simulink model "AUAV_V3_TestSensors"  (R2015a)
settings: Solver=FixedStepDiscrete  StartTime=0.0  StopTime=10.0  FixedStep=T  RelTol=1e-3
PreLoadFcn:
  | %T = 0.0025;
  | MavlinkBus;
  | mcuInit;
  | % Baro Altitude Computation
  | % =========================
  | basePressure = 98192.64;
  | baseTemp = 288.215;
  | lapseRate = -0.00198122;
  | baseHeight = 0;
values from neighbouring files (symbols this model uses):
  apSampleTime = 0.01    [mcuInit.m]
  latlong_WP = 1    [mcuInit.m]
  mavlink_attitude_t = Simulink.Bus    [MavlinkBusMarcello.m]
  mavlink_gps_raw_int_t = Simulink.Bus    [MavlinkBus.m]    (also in MavlinkBusMarcello.m)
  mavlink_raw_imu_t = Simulink.Bus    [MavlinkBus.m]    (also in MavlinkBusMarcello.m)
  mavlink_scaled_pressure_t = Simulink.Bus    [MavlinkBus.m]    (also in MavlinkBusMarcello.m)
  mavlink_servo_output_raw_t = Simulink.Bus    [MavlinkBusMarcello.m]
  mavlink_slugs_navigation_t = Simulink.Bus    [MavlinkBusMarcello.m]
  mavlink_sys_status_t = Simulink.Bus    [MavlinkBus.m]    (also in MavlinkBusMarcello.m)
  T = 0.01    [mcuInit.m]
  Xpoints = [0 0]    [mcuInit.m]
  Ypoints = [0 0]    [mcuInit.m]
  Zpoints = [0 0]    [mcuInit.m]
undefined symbols (not defined in the file or in its folder): A0, A14, A15, A2, A3, A4, A5, A6, accBiasRateLimit, B0, bankCommandLimit, barAdjust, baroCutoff, baroCutTemp, cubeAccelGain16405, cubeGyroGain16405, cubeMagGain16405, D0, D11, D7, D8, daLimit, data, daTrimMax, daTrimMin, deLimit, deTrimMax, deTrimMin, drLimit, drTrimMax, drTrimMin, dtLimit, dtTrimMax, dtTrimMin, F2, F3, G0, G13, G15, gaind, GS_location, gyroBiasRateLimit, IC1max, IPStar, ISA_g, Max, maxAcc, MaxDwnPthStar, maxDynPressure, maxEta, mlParamInterface, ms, OC1max, P112, P125, P127, P16, P20, P21, P30 ... (+26)
undefined symbols (not defined in the file): baroOffset, baroScale, barTGain1, barTGain2, barTMean1, barTMean2, bda, bde, bdr, bdt, bICda, bICde, bICdr, bICdt, derivativesConstant, lowRateSensorCutoff, mainSensorCutoff, mda, mde, mdr, mdt, mICda, mICde, mICdr, mICdt, pitotOffset, pitotScale, pitTGain1, pitTGain2, pitTMean1, pitTMean2, powerOffset, powerScale, pressureSensorCutoff, tempOffset, tempScale, vzCutoff, xCutoff, yCutoff
libraries: MCHP_Blockset x158, simulink x84, SLUGS_Library x31, aerolibconvert2 x6, aerolibutil x4, aerolibtransform2 x3, dspmtrx3 x2, aerolibobsolete x2
(part 22 of 24)

== system AUAV_V3_TestSensors/Inner Loop// Navigation/Lateral Channel Encaps [updated 4.28.16]/Lateral Channel/Roll Control [PID]/Trapezoidal Integrator/Protect NaNs  ==
  In1 : Inport
  Integer Delay3 : Delay  DelayLength=1  InputProcessing=Inherited  SampleTime=T
  Relational Operator2 : RelationalOperator  Operator===  OutDataTypeStr=uint(8)
  Switch3 : Switch  Criteria=u2 > Threshold  Threshold=0.3  SampleTime=.01
  Out1 : Outport
  wires:
  Integer Delay3/1 -> Switch3/3
  Switch3/1 -> Out1/1, Integer Delay3/1
  In1/1 -> Relational Operator2/2, Relational Operator2/1, Switch3/1
  Relational Operator2/1 -> Switch3/2

== system AUAV_V3_TestSensors/Inner Loop// Navigation/Lateral Channel Encaps [updated 4.28.16]/Lateral Channel/Roll Control [PID]/Trapezoidal Integrator/Protect NaNs1 ==
  In1 : Inport
  Integer Delay3 : Delay  DelayLength=1  InputProcessing=Inherited  SampleTime=T
  Relational Operator2 : RelationalOperator  Operator===  OutDataTypeStr=uint(8)
  Switch3 : Switch  Criteria=u2 > Threshold  Threshold=0.3  SampleTime=.01
  Out1 : Outport
  wires:
  Integer Delay3/1 -> Switch3/3
  Switch3/1 -> Out1/1, Integer Delay3/1
  In1/1 -> Relational Operator2/2, Relational Operator2/1, Switch3/1
  Relational Operator2/1 -> Switch3/2

== system AUAV_V3_TestSensors/Inner Loop// Navigation/Lateral Channel Encaps [updated 4.28.16]/Lateral Channel/Sideslip Compensation/Bank to Psi Dot/dsPIC_tan ==
  x : Inport
  Environment Controller : simulink/Signal Routing/Environment Controller
  Trigonometric Function : Trigonometry  Operator=tan
  myTan() apUtils.c [updated 5.1.16] : MCHP_Blockset/User Functions/C Function Call  ParseFilesChkbx=off  ListFunctions1=Custom Function  Function1=float myTan(float x)  AddHeaderDeclaration=on  Function1Type=when block is updated (default)  Fct1BlockIn=x  FctReturnBlockOut=on  ORDERING=None  SampleTime=-1  MCHP_MASTERLINK=|  PinDigitalInput=[]  PinDigitalOutput=[]  PinAnalogInput=[]
      | AUAV_V3_TestSensors/Microchip Master
      | AUAV V3 Board
      | Busy Flag on D2 (RA6)
  tan(x) : Outport
  wires:
  Environment Controller/1 -> tan(x)/1
  Trigonometric Function/1 -> Environment Controller/1
  x/1 -> Trigonometric Function/1, myTan() apUtils.c [updated 5.1.16]/1
  myTan() apUtils.c [updated 5.1.16]/1 -> Environment Controller/2

== system AUAV_V3_TestSensors/Inner Loop// Navigation/Lateral Channel Encaps [updated 4.28.16]/Lateral Channel/Sideslip Compensation/Low Pass/Compute Coef ==
  a : Inport
  Enable : EnablePort
  -T : Gain  Gain=-apSampleTime  SampleTime=apSampleTime
  1-c : Sum  Inputs=-+  OutDataTypeStr=single  SampleTime=apSampleTime
  Constant : Constant
  Math Function : Math  SaturateOnIntegerOverflow=on
  b : Outport
  c : Outport  Port=2
  wires:
  -T/1 -> Math Function/1
  Math Function/1 -> 1-c/1, c/1  "c"
  Constant/1 -> 1-c/2
  1-c/1 -> b/1
  a/1 -> -T/1

== system AUAV_V3_TestSensors/Inner Loop// Navigation/Lateral Channel Encaps [updated 4.28.16]/Lateral Channel/Sideslip Compensation/Low Pass/Detect Change ==
  Data : Inport
  Abs1 : Abs  SampleTime=apSampleTime
  Difference1 : simulink/Discrete/Difference  ICPrevInput=0.0  InputProcessing=Inherited  OutMin=[]  OutMax=[]  OutDataType=sfix(16)  OutScaling=2^-10  DoSatur=off
  Saturation1 : Saturate  UpperLimit=1  LowerLimit=0  SampleTime=apSampleTime
  change? : Outport
  wires:
  Difference1/1 -> Abs1/1
  Abs1/1 -> Saturation1/1
  Data/1 -> Difference1/1
  Saturation1/1 -> change?/1

== system AUAV_V3_TestSensors/Inner Loop// Navigation/Lateral Channel Encaps [updated 4.28.16]/Lateral Channel/Sideslip Compensation/psi_dot to Bank/dsPIC_atan ==
  x : Inport
  Environment Controller : simulink/Signal Routing/Environment Controller
  Trigonometric Function : Trigonometry  Operator=atan
  myTan() apUtils.c [updated 5.1.16] : MCHP_Blockset/User Functions/C Function Call  ParseFilesChkbx=off  ListFunctions1=Custom Function  Function1=float myTan(float x)  AddHeaderDeclaration=on  Function1Type=when block is updated (default)  Fct1BlockIn=x  FctReturnBlockOut=on  ORDERING=None  SampleTime=-1  MCHP_MASTERLINK=|  PinDigitalInput=[]  PinDigitalOutput=[]  PinAnalogInput=[]
      | AUAV_V3_TestSensors/Microchip Master
      | AUAV V3 Board
      | Busy Flag on D2 (RA6)
  atan(x) : Outport
  wires:
  x/1 -> Trigonometric Function/1, myTan() apUtils.c [updated 5.1.16]/1
  Trigonometric Function/1 -> Environment Controller/1
  Environment Controller/1 -> atan(x)/1
  myTan() apUtils.c [updated 5.1.16]/1 -> Environment Controller/2

== system AUAV_V3_TestSensors/Inner Loop// Navigation/Lateral Channel Encaps [updated 4.28.16]/Lateral Channel/Yaw Damper [PID]/Trapezoidal Integrator/Protect NaNs  ==
  In1 : Inport
  Integer Delay3 : Delay  DelayLength=1  InputProcessing=Inherited  SampleTime=T
  Relational Operator2 : RelationalOperator  Operator===  OutDataTypeStr=uint(8)
  Switch3 : Switch  Criteria=u2 > Threshold  Threshold=0.3  SampleTime=.01
  Out1 : Outport
  wires:
  Integer Delay3/1 -> Switch3/3
  Switch3/1 -> Out1/1, Integer Delay3/1
  In1/1 -> Relational Operator2/2, Relational Operator2/1, Switch3/1
  Relational Operator2/1 -> Switch3/2

== system AUAV_V3_TestSensors/Inner Loop// Navigation/Lateral Channel Encaps [updated 4.28.16]/Lateral Channel/Yaw Damper [PID]/Trapezoidal Integrator/Protect NaNs1 ==
  In1 : Inport
  Integer Delay3 : Delay  DelayLength=1  InputProcessing=Inherited  SampleTime=T
  Relational Operator2 : RelationalOperator  Operator===  OutDataTypeStr=uint(8)
  Switch3 : Switch  Criteria=u2 > Threshold  Threshold=0.3  SampleTime=.01
  Out1 : Outport
  wires:
  Integer Delay3/1 -> Switch3/3
  Switch3/1 -> Out1/1, Integer Delay3/1
  In1/1 -> Relational Operator2/2, Relational Operator2/1, Switch3/1
  Relational Operator2/1 -> Switch3/2

== system AUAV_V3_TestSensors/Inner Loop// Navigation/Longitudinal Channel Encaps [updated 4.28.16]/Longitudinal Channel/Airspeed Hold [PID]/Trapezoidal Integrator/Protect NaNs  ==
  In1 : Inport
  Integer Delay3 : Delay  DelayLength=1  InputProcessing=Inherited  SampleTime=T
  Relational Operator2 : RelationalOperator  Operator===  OutDataTypeStr=uint(8)
  Switch3 : Switch  Criteria=u2 > Threshold  Threshold=0.3  SampleTime=.01
  Out1 : Outport
  wires:
  Integer Delay3/1 -> Switch3/3
  Switch3/1 -> Out1/1, Integer Delay3/1
  In1/1 -> Relational Operator2/2, Relational Operator2/1, Switch3/1
  Relational Operator2/1 -> Switch3/2

== system AUAV_V3_TestSensors/Inner Loop// Navigation/Longitudinal Channel Encaps [updated 4.28.16]/Longitudinal Channel/Airspeed Hold [PID]/Trapezoidal Integrator/Protect NaNs1 ==
  In1 : Inport
  Integer Delay3 : Delay  DelayLength=1  InputProcessing=Inherited  SampleTime=T
  Relational Operator2 : RelationalOperator  Operator===  OutDataTypeStr=uint(8)
  Switch3 : Switch  Criteria=u2 > Threshold  Threshold=0.3  SampleTime=.01
  Out1 : Outport
  wires:
  Integer Delay3/1 -> Switch3/3
  Switch3/1 -> Out1/1, Integer Delay3/1
  In1/1 -> Relational Operator2/2, Relational Operator2/1, Switch3/1
  Relational Operator2/1 -> Switch3/2

== system AUAV_V3_TestSensors/Inner Loop// Navigation/Longitudinal Channel Encaps [updated 4.28.16]/Longitudinal Channel/Height Error to Pitch Command [PI]/Trapezoidal Integrator/Protect NaNs ==
  In1 : Inport
  Integer Delay3 : Delay  DelayLength=1  InputProcessing=Inherited  SampleTime=T
  Relational Operator2 : RelationalOperator  Operator===  OutDataTypeStr=uint(8)
  Switch3 : Switch  Criteria=u2 > Threshold  Threshold=0.3  SampleTime=.01
  Out1 : Outport
  wires:
  Integer Delay3/1 -> Switch3/3
  Switch3/1 -> Out1/1, Integer Delay3/1
  In1/1 -> Relational Operator2/2, Relational Operator2/1, Switch3/1
  Relational Operator2/1 -> Switch3/2

== system AUAV_V3_TestSensors/Inner Loop// Navigation/Longitudinal Channel Encaps [updated 4.28.16]/Longitudinal Channel/Height Error to Pitch Command [PI]/Trapezoidal Integrator/Protect NaNs  ==
  In1 : Inport
  Integer Delay3 : Delay  DelayLength=1  InputProcessing=Inherited  SampleTime=T
  Relational Operator2 : RelationalOperator  Operator===  OutDataTypeStr=uint(8)
  Switch3 : Switch  Criteria=u2 > Threshold  Threshold=0.3  SampleTime=.01
  Out1 : Outport
  wires:
  Integer Delay3/1 -> Switch3/3
  Switch3/1 -> Out1/1, Integer Delay3/1
  In1/1 -> Relational Operator2/2, Relational Operator2/1, Switch3/1
  Relational Operator2/1 -> Switch3/2

== system AUAV_V3_TestSensors/Inner Loop// Navigation/Longitudinal Channel Encaps [updated 4.28.16]/Longitudinal Channel/Pitch To Elevator [PID]/Trapezoidal Integrator/Protect NaNs  ==
  In1 : Inport
  Integer Delay3 : Delay  DelayLength=1  InputProcessing=Inherited  SampleTime=T
  Relational Operator2 : RelationalOperator  Operator===  OutDataTypeStr=uint(8)
  Switch3 : Switch  Criteria=u2 > Threshold  Threshold=0.3  SampleTime=.01
  Out1 : Outport
  wires:
  Integer Delay3/1 -> Switch3/3
  Switch3/1 -> Out1/1, Integer Delay3/1
  In1/1 -> Relational Operator2/2, Relational Operator2/1, Switch3/1
  Relational Operator2/1 -> Switch3/2

== system AUAV_V3_TestSensors/Inner Loop// Navigation/Longitudinal Channel Encaps [updated 4.28.16]/Longitudinal Channel/Pitch To Elevator [PID]/Trapezoidal Integrator/Protect NaNs1 ==
  In1 : Inport
  Integer Delay3 : Delay  DelayLength=1  InputProcessing=Inherited  SampleTime=T
  Relational Operator2 : RelationalOperator  Operator===  OutDataTypeStr=uint(8)
  Switch3 : Switch  Criteria=u2 > Threshold  Threshold=0.3  SampleTime=.01
  Out1 : Outport
  wires:
  Integer Delay3/1 -> Switch3/3
  Switch3/1 -> Out1/1, Integer Delay3/1
  In1/1 -> Relational Operator2/2, Relational Operator2/1, Switch3/1
  Relational Operator2/1 -> Switch3/2

== system AUAV_V3_TestSensors/Inner Loop// Navigation/Longitudinal Channel Encaps [updated 4.28.16]/Longitudinal Channel/Pitot Control End/Air Density from Height/dsPIC Power ==
  u : Inport
  v : Inport  Port=2
  Environment Controller : simulink/Signal Routing/Environment Controller
  Math Function : Math  Operator=pow  SaturateOnIntegerOverflow=on
  myPow() apUtils.c [updated 5.1.16] : MCHP_Blockset/User Functions/C Function Call  ParseFilesChkbx=off  ListFunctions1=Custom Function  Function1=float myPow(float x, float toTheN)  AddHeaderDeclaration=on  Function1Type=when block is updated (default)  Fct1BlockIn="x  , toTheN"  FctReturnBlockOut=on  ORDERING=None  SampleTime=-1  MCHP_MASTERLINK=|  PinDigitalInput=[]  PinDigitalOutput=[]  PinAnalogInput=[]
      | AUAV_V3_TestSensors/Microchip Master
      | AUAV V3 Board
      | Busy Flag on D2 (RA6)
  u^v : Outport
  wires:
  Environment Controller/1 -> u^v/1
  Math Function/1 -> Environment Controller/1
  v/1 -> Math Function/2, myPow() apUtils.c [updated 5.1.16]/2
  u/1 -> Math Function/1, myPow() apUtils.c [updated 5.1.16]/1
  myPow() apUtils.c [updated 5.1.16]/1 -> Environment Controller/2

== system AUAV_V3_TestSensors/Inner Loop// Navigation/Longitudinal Channel Encaps [updated 4.28.16]/Longitudinal Channel/Pitot Control End/Compute Airspeed/dsPIC_SQRT ==
  x : Inport
  Environment Controller : simulink/Signal Routing/Environment Controller
  Math Function1 : Math  Operator=sqrt  SaturateOnIntegerOverflow=on
  mySqrt() apUtils.c [updated 5.1.16] : MCHP_Blockset/User Functions/C Function Call  ParseFilesChkbx=off  ListFunctions1=Custom Function  Function1=float mySqrt(float x)  AddHeaderDeclaration=off  Function1Type=when block is updated (default)  Fct1BlockIn=x  FctReturnBlockOut=on  DataCollected=0  ORDERING=None  SampleTime=-1  MCHP_MASTERLINK=|  PinDigitalInput=[]  PinDigitalOutput=[]  PinAnalogInput=[]
      | AUAV_V3_TestSensors/Microchip Master
      | AUAV V3 Board
      | Busy Flag on D2 (RA6)
  negprotect : MATLAB Function  TreatAsAtomicUnit=on
  sqrt(x) : Outport
  wires:
  x/1 -> negprotect/1(val)
  negprotect/1(zpVal) -> Math Function1/1, mySqrt() apUtils.c [updated 5.1.16]/1
  Environment Controller/1 -> sqrt(x)/1
  Math Function1/1 -> Environment Controller/1
  mySqrt() apUtils.c [updated 5.1.16]/1 -> Environment Controller/2

== system AUAV_V3_TestSensors/Inner Loop// Navigation/Navigation Encaps [updated 4.28.16]/Navigation/Circle Navigation/Intersection. Circular Navigation/Compute Angle Between Vectors1 ==
  Vxyz : Inport
  |Vg| : Inport  Port=2
  P3 : Inport  Port=3
  Product8 : Product  Inputs=*/  RndMeth=Zero
  Product9 : Product  RndMeth=Zero
  Vector Norm : Subsystem  AncestorBlock=SLUGS_Library/Vector Norm
  "[-1 1]" : Saturate  UpperLimit=1  LowerLimit=-1
  dsPIC Dot Product : SLUGS_Library/dsPIC Dot Product
  dsPIC_acos : Subsystem  AncestorBlock=SLUGS_Library/dsPIC_acos
  negprotect3 : MATLAB Function  TreatAsAtomicUnit=on
  alpha : Outport
  wires:
  dsPIC_acos/1(acos(x)) -> alpha/1
  negprotect3/1(zpVal) -> Product8/2
  "[-1 1]"/1 -> dsPIC_acos/1(x)
  Product8/1 -> "[-1 1]"/1
  Product9/1 -> negprotect3/1(val)
  |Vg|/1 -> Product9/2
  Vector Norm/1(Norm) -> Product9/1
  dsPIC Dot Product/1 -> Product8/1
  Vxyz/1 -> dsPIC Dot Product/1
  P3/1 -> Vector Norm/1(Vector), dsPIC Dot Product/2

== system AUAV_V3_TestSensors/Inner Loop// Navigation/Navigation Encaps [updated 4.28.16]/Navigation/Circle Navigation/Intersection. Circular Navigation/Compute Angle Between Vectors2 ==
  Vxyz : Inport
  |Vg| : Inport  Port=2
  P3 : Inport  Port=3
  Product8 : Product  Inputs=*/  RndMeth=Zero
  Product9 : Product  RndMeth=Zero
  Vector Norm : Subsystem  AncestorBlock=SLUGS_Library/Vector Norm
  "[-1 1]" : Saturate  UpperLimit=1  LowerLimit=-1
  dsPIC Dot Product : SLUGS_Library/dsPIC Dot Product
  dsPIC_acos : Subsystem  AncestorBlock=SLUGS_Library/dsPIC_acos
  negprotect3 : MATLAB Function  TreatAsAtomicUnit=on
  alpha : Outport
  wires:
  dsPIC_acos/1(acos(x)) -> alpha/1
  negprotect3/1(zpVal) -> Product8/2
  "[-1 1]"/1 -> dsPIC_acos/1(x)
  Product8/1 -> "[-1 1]"/1
  Product9/1 -> negprotect3/1(val)
  |Vg|/1 -> Product9/2
  Vector Norm/1(Norm) -> Product9/1
  dsPIC Dot Product/1 -> Product8/1
  Vxyz/1 -> dsPIC Dot Product/1
  P3/1 -> Vector Norm/1(Vector), dsPIC Dot Product/2

== system AUAV_V3_TestSensors/Inner Loop// Navigation/Navigation Encaps [updated 4.28.16]/Navigation/Circle Navigation/Intersection. Circular Navigation/dsPIC_ABS ==
  x : Inport
  Abs : Abs
  Environment Controller : simulink/Signal Routing/Environment Controller
  myAbs() apUtils.c [updated 5.1.16] : MCHP_Blockset/User Functions/C Function Call  ParseFilesChkbx=off  ListFunctions1=Custom Function  Function1=float myAbs(float x)  AddHeaderDeclaration=off  Function1Type=when block is updated (default)  Fct1BlockIn=x  FctReturnBlockOut=on  DataCollected=0  ORDERING=None  SampleTime=-1  MCHP_MASTERLINK=|  PinDigitalInput=[]  PinDigitalOutput=[]  PinAnalogInput=[]
      | AUAV_V3_TestSensors/Microchip Master
      | AUAV V3 Board
      | Busy Flag on D2 (RA6)
  |x| : Outport
  wires:
  Environment Controller/1 -> |x|/1
  Abs/1 -> Environment Controller/1
  myAbs() apUtils.c [updated 5.1.16]/1 -> Environment Controller/2
  x/1 -> Abs/1, myAbs() apUtils.c [updated 5.1.16]/1

== system AUAV_V3_TestSensors/Inner Loop// Navigation/Navigation Encaps [updated 4.28.16]/Navigation/Circle Navigation/Intersection. Circular Navigation/dsPIC_ABS1 ==
  x : Inport
  Abs : Abs
  Environment Controller : simulink/Signal Routing/Environment Controller
  myAbs() apUtils.c [updated 5.1.16] : MCHP_Blockset/User Functions/C Function Call  ParseFilesChkbx=off  ListFunctions1=Custom Function  Function1=float myAbs(float x)  AddHeaderDeclaration=off  Function1Type=when block is updated (default)  Fct1BlockIn=x  FctReturnBlockOut=on  DataCollected=0  ORDERING=None  SampleTime=-1  MCHP_MASTERLINK=|  PinDigitalInput=[]  PinDigitalOutput=[]  PinAnalogInput=[]
      | AUAV_V3_TestSensors/Microchip Master
      | AUAV V3 Board
      | Busy Flag on D2 (RA6)
  |x| : Outport
  wires:
  Environment Controller/1 -> |x|/1
  Abs/1 -> Environment Controller/1
  myAbs() apUtils.c [updated 5.1.16]/1 -> Environment Controller/2
  x/1 -> Abs/1, myAbs() apUtils.c [updated 5.1.16]/1

== system AUAV_V3_TestSensors/Inner Loop// Navigation/Navigation Encaps [updated 4.28.16]/Navigation/Circle Navigation/Intersection. Circular Navigation/dsPIC_SQRT ==
  x : Inport
  Environment Controller : simulink/Signal Routing/Environment Controller
  Math Function1 : Math  Operator=sqrt  SaturateOnIntegerOverflow=on
  mySqrt() apUtils.c [updated 5.1.16] : MCHP_Blockset/User Functions/C Function Call  ParseFilesChkbx=off  ListFunctions1=Custom Function  Function1=float mySqrt(float x)  AddHeaderDeclaration=off  Function1Type=when block is updated (default)  Fct1BlockIn=x  FctReturnBlockOut=on  DataCollected=0  ORDERING=None  SampleTime=-1  MCHP_MASTERLINK=|  PinDigitalInput=[]  PinDigitalOutput=[]  PinAnalogInput=[]
      | AUAV_V3_TestSensors/Microchip Master
      | AUAV V3 Board
      | Busy Flag on D2 (RA6)
  negprotect : MATLAB Function  TreatAsAtomicUnit=on
  sqrt(x) : Outport
  wires:
  x/1 -> negprotect/1(val)
  negprotect/1(zpVal) -> Math Function1/1, mySqrt() apUtils.c [updated 5.1.16]/1
  Environment Controller/1 -> sqrt(x)/1
  Math Function1/1 -> Environment Controller/1
  mySqrt() apUtils.c [updated 5.1.16]/1 -> Environment Controller/2

== system AUAV_V3_TestSensors/Inner Loop// Navigation/Navigation Encaps [updated 4.28.16]/Navigation/Circle Navigation/Vector Norm/dsPIC_SQRT ==
  x : Inport
  Environment Controller : simulink/Signal Routing/Environment Controller
  Math Function1 : Math  Operator=sqrt  SaturateOnIntegerOverflow=on
  mySqrt() apUtils.c [updated 5.1.16] : MCHP_Blockset/User Functions/C Function Call  ParseFilesChkbx=off  ListFunctions1=Custom Function  Function1=float mySqrt(float x)  AddHeaderDeclaration=off  Function1Type=when block is updated (default)  Fct1BlockIn=x  FctReturnBlockOut=on  DataCollected=0  ORDERING=None  SampleTime=-1  MCHP_MASTERLINK=|  PinDigitalInput=[]  PinDigitalOutput=[]  PinAnalogInput=[]
      | AUAV_V3_TestSensors/Microchip Master
      | AUAV V3 Board
      | Busy Flag on D2 (RA6)
  negprotect : MATLAB Function  TreatAsAtomicUnit=on
  sqrt(x) : Outport
  wires:
  x/1 -> negprotect/1(val)
  negprotect/1(zpVal) -> Math Function1/1, mySqrt() apUtils.c [updated 5.1.16]/1
  Environment Controller/1 -> sqrt(x)/1
  Math Function1/1 -> Environment Controller/1
  mySqrt() apUtils.c [updated 5.1.16]/1 -> Environment Controller/2

== system AUAV_V3_TestSensors/Inner Loop// Navigation/Navigation Encaps [updated 4.28.16]/Navigation/Get 2D Groundspeed/Vector Norm/dsPIC_SQRT ==
  x : Inport
  Environment Controller : simulink/Signal Routing/Environment Controller
  Math Function1 : Math  Operator=sqrt  SaturateOnIntegerOverflow=on
  mySqrt() apUtils.c [updated 5.1.16] : MCHP_Blockset/User Functions/C Function Call  ParseFilesChkbx=off  ListFunctions1=Custom Function  Function1=float mySqrt(float x)  AddHeaderDeclaration=on  Function1Type=when block is updated (default)  Fct1BlockIn=x  FctReturnBlockOut=on  DataCollected=0  ORDERING=None  SampleTime=-1  MCHP_MASTERLINK=|  PinDigitalInput=[]  PinDigitalOutput=[]  PinAnalogInput=[]
      | AUAV_V3_TestSensors/Microchip Master
      | AUAV V3 Board
      | Busy Flag on D2 (RA6)
  negprotect : MATLAB Function  TreatAsAtomicUnit=on
  sqrt(x) : Outport
  wires:
  x/1 -> negprotect/1(val)
  negprotect/1(zpVal) -> Math Function1/1, mySqrt() apUtils.c [updated 5.1.16]/1
  Environment Controller/1 -> sqrt(x)/1
  Math Function1/1 -> Environment Controller/1
  mySqrt() apUtils.c [updated 5.1.16]/1 -> Environment Controller/2

== system AUAV_V3_TestSensors/Inner Loop// Navigation/Navigation Encaps [updated 4.28.16]/Navigation/L2+/Get Sin, Cos eta/2D Dot Product  ==
  Vxyz : Inport
  L2_vec : Inport  Port=2
  Demux : Demux  Outputs=3
  Demux1 : Demux  Outputs=3
  Product : Product  RndMeth=Zero
  Product1 : Product  RndMeth=Zero
  Subtract : Sum  Inputs=2
  Terminator : Terminator
  Terminator1 : Terminator
  2D _dot : Outport
  wires:
  Demux/2 -> Product1/2
  Demux1/2 -> Product1/1
  Demux/1 -> Product/2
  Demux1/1 -> Product/1
  Demux/3 -> Terminator/1
  Demux1/3 -> Terminator1/1
  Product/1 -> Subtract/1
  Product1/1 -> Subtract/2
  L2_vec/1 -> Demux1/1
  Subtract/1 -> 2D _dot/1
  Vxyz/1 -> Demux/1

== system AUAV_V3_TestSensors/Inner Loop// Navigation/Navigation Encaps [updated 4.28.16]/Navigation/L2+/Get Sin, Cos eta/Get Groundspeed ==
  L2_vec : Inport  SampleTime=apSampleTime
  Vector Norm : Subsystem  AncestorBlock=SLUGS_Library/Vector Norm
  Zero out Z1 : MATLAB Function  TreatAsAtomicUnit=on
  |L2| : Outport
  wires:
  Vector Norm/1(Norm) -> |L2|/1
  Zero out Z1/1(P) -> Vector Norm/1(Vector)
  L2_vec/1 -> Zero out Z1/1(Pin)

== system AUAV_V3_TestSensors/Inner Loop// Navigation/Navigation Encaps [updated 4.28.16]/Navigation/L2+/Get Sin, Cos eta/Get ZProd ==
  L2_vec : Inport
  Vxyz : Inport  Port=2
  Demux : Demux  Outputs=3
  Demux1 : Demux  Outputs=3
  Product : Product  RndMeth=Zero
  Product1 : Product  RndMeth=Zero
  Subtract : Sum  Inputs=+-
  Terminator : Terminator
  Terminator1 : Terminator
  Z_prod : Outport
  wires:
  Vxyz/1 -> Demux/1
  Subtract/1 -> Z_prod/1
  L2_vec/1 -> Demux1/1
  Product1/1 -> Subtract/2
  Product/1 -> Subtract/1
  Demux1/1 -> Product1/1
  Demux/2 -> Product1/2
  Demux1/2 -> Product/1
  Demux/1 -> Product/2
  Demux1/3 -> Terminator1/1
  Demux/3 -> Terminator/1

== system AUAV_V3_TestSensors/Inner Loop// Navigation/Navigation Encaps [updated 4.28.16]/Navigation/L2+/Subsystem/dsPIC_atan ==
  x : Inport
  Environment Controller : simulink/Signal Routing/Environment Controller
  Trigonometric Function : Trigonometry  Operator=atan
  myAtan() apUtils.c [updated 5.1.16] : MCHP_Blockset/User Functions/C Function Call  ParseFilesChkbx=off  ListFunctions1=Custom Function  Function1=float myAtan(float x)  AddHeaderDeclaration=on  Function1Type=when block is updated (default)  Fct1BlockIn=x  FctReturnBlockOut=on  DataCollected=0  ORDERING=None  SampleTime=-1  MCHP_MASTERLINK=|  PinDigitalInput=[]  PinDigitalOutput=[]  PinAnalogInput=[]
      | AUAV_V3_TestSensors/Microchip Master
      | AUAV V3 Board
      | Busy Flag on D2 (RA6)
  atan(x) : Outport
  wires:
  x/1 -> Trigonometric Function/1, myAtan() apUtils.c [updated 5.1.16]/1
  Trigonometric Function/1 -> Environment Controller/1
  myAtan() apUtils.c [updated 5.1.16]/1 -> Environment Controller/2
  Environment Controller/1 -> atan(x)/1

== system AUAV_V3_TestSensors/Inner Loop// Navigation/Navigation Encaps [updated 4.28.16]/Navigation/Line Segment/Vector Norm/dsPIC_SQRT ==
  x : Inport
  Environment Controller : simulink/Signal Routing/Environment Controller
  Math Function1 : Math  Operator=sqrt  SaturateOnIntegerOverflow=on
  mySqrt() apUtils.c [updated 5.1.16] : MCHP_Blockset/User Functions/C Function Call  ParseFilesChkbx=off  ListFunctions1=Custom Function  Function1=float mySqrt(float x)  AddHeaderDeclaration=on  Function1Type=when block is updated (default)  Fct1BlockIn=x  FctReturnBlockOut=on  DataCollected=0  ORDERING=None  SampleTime=-1  MCHP_MASTERLINK=|  PinDigitalInput=[]  PinDigitalOutput=[]  PinAnalogInput=[]
      | AUAV_V3_TestSensors/Microchip Master
      | AUAV V3 Board
      | Busy Flag on D2 (RA6)
  negprotect : MATLAB Function  TreatAsAtomicUnit=on
  sqrt(x) : Outport
  wires:
  x/1 -> negprotect/1(val)
  negprotect/1(zpVal) -> Math Function1/1, mySqrt() apUtils.c [updated 5.1.16]/1
  Environment Controller/1 -> sqrt(x)/1
  Math Function1/1 -> Environment Controller/1
  mySqrt() apUtils.c [updated 5.1.16]/1 -> Environment Controller/2

== system AUAV_V3_TestSensors/Inner Loop// Navigation/Navigation Encaps [updated 4.28.16]/Navigation/Normal WP Navigation/Compute WP Switching Trigger/Compute Projection ==
  Pned : Inport
  ToWp : Inport  Port=2
  T : Inport  Port=3
  Protect NaNs : Subsystem
  Subtract : Sum  Inputs=-+  OutDataTypeStr=single
  dsPIC Dot Product : SLUGS_Library/dsPIC Dot Product
  D2wp1 : Outport
  wires:
  dsPIC Dot Product/1 -> Protect NaNs/1(In1)
  T/1 -> dsPIC Dot Product/2
  Subtract/1 -> dsPIC Dot Product/1
  ToWp/1 -> Subtract/2
  Pned/1 -> Subtract/1
  Protect NaNs/1(Out1) -> D2wp1/1

== system AUAV_V3_TestSensors/Inner Loop// Navigation/Navigation Encaps [updated 4.28.16]/Navigation/Normal WP Navigation/Compute WP Switching Trigger/dsPIC_ABS ==
  x : Inport
  Abs : Abs
  Environment Controller : simulink/Signal Routing/Environment Controller
  myAbs() apUtils.c [updated 5.1.16] : MCHP_Blockset/User Functions/C Function Call  ParseFilesChkbx=off  ListFunctions1=Custom Function  Function1=float myAbs(float x)  AddHeaderDeclaration=on  Function1Type=when block is updated (default)  Fct1BlockIn=x  FctReturnBlockOut=on  DataCollected=0  ORDERING=None  SampleTime=-1  MCHP_MASTERLINK=|  PinDigitalInput=[]  PinDigitalOutput=[]  PinAnalogInput=[]
      | AUAV_V3_TestSensors/Microchip Master
      | AUAV V3 Board
      | Busy Flag on D2 (RA6)
  |x| : Outport
  wires:
  x/1 -> Abs/1, myAbs() apUtils.c [updated 5.1.16]/1
  Environment Controller/1 -> |x|/1
  myAbs() apUtils.c [updated 5.1.16]/1 -> Environment Controller/2
  Abs/1 -> Environment Controller/1

== system AUAV_V3_TestSensors/Inner Loop// Navigation/Navigation Encaps [updated 4.28.16]/Navigation/Normal WP Navigation/Compute WP Switching Trigger/dsPIC_SQRT ==
  x : Inport
  Environment Controller : simulink/Signal Routing/Environment Controller
  Math Function1 : Math  Operator=sqrt  SaturateOnIntegerOverflow=on
  mySqrt() apUtils.c [updated 5.1.16] : MCHP_Blockset/User Functions/C Function Call  ParseFilesChkbx=off  ListFunctions1=Custom Function  Function1=float mySqrt(float x)  AddHeaderDeclaration=on  Function1Type=when block is updated (default)  Fct1BlockIn=x  FctReturnBlockOut=on  DataCollected=0  ORDERING=None  SampleTime=-1  MCHP_MASTERLINK=|  PinDigitalInput=[]  PinDigitalOutput=[]  PinAnalogInput=[]
      | AUAV_V3_TestSensors/Microchip Master
      | AUAV V3 Board
      | Busy Flag on D2 (RA6)
  negprotect : MATLAB Function  TreatAsAtomicUnit=on
  sqrt(x) : Outport
  wires:
  x/1 -> negprotect/1(val)
  negprotect/1(zpVal) -> Math Function1/1, mySqrt() apUtils.c [updated 5.1.16]/1
  Environment Controller/1 -> sqrt(x)/1
  Math Function1/1 -> Environment Controller/1
  mySqrt() apUtils.c [updated 5.1.16]/1 -> Environment Controller/2

== system AUAV_V3_TestSensors/Inner Loop// Navigation/Navigation Encaps [updated 4.28.16]/Navigation/Normal WP Navigation/Get Frenet/Compute Frenet ==
  Pos 1 : Inport
  Pos 2 : Inport  Port=2
  Add : Sum  Inputs=-+
  Normalize Vector : Subsystem  AncestorBlock=SLUGS_Library/Navigation/Normalize Vector
  "Normalize Vector " : Subsystem  AncestorBlock=SLUGS_Library/Navigation/Normalize Vector
  Select N Terms : MATLAB Function  TreatAsAtomicUnit=on
  T : Outport
  N : Outport  Port=2
  wires:
  "Normalize Vector "/1(Normalized) -> N/1
  Select N Terms/1(N) -> "Normalize Vector "/1(Vector)
  Normalize Vector/1(Normalized) -> Select N Terms/1(T), T/1
  Add/1 -> Normalize Vector/1(Vector)
  Pos 2/1 -> Add/2
  Pos 1/1 -> Add/1

== system AUAV_V3_TestSensors/Inner Loop// Navigation/Navigation Encaps [updated 4.28.16]/Navigation/Normal WP Navigation/Get Frenet/get WP Coord from Index1 ==
  WP Idx : Inport
  GS LLA : Inport  Port=2
  GS R_in : Inport  Port=3
  Demux1 : Demux  Outputs=3
  Environment Controller1 : simulink/Signal Routing/Environment Controller
  Geod2LTP2 : SLUGS_Library/Navigation/Geod2LTP
  Get WP Coord navsupport.c [updated 5.1.16] : MCHP_Blockset/User Functions/C Function Call  ParseFilesChkbx=off  ListFunctions1=Custom Function  Function1=void getWP(unsigned char idx, float* WPpos)  AddHeaderDeclaration=on  Function1Type=when block is updated (default)  Fct1BlockIn=idx  FctReturnBlockOut=on  Fct1BlockOut=WPpos[3]  DataCollected=0  ORDERING=None  SampleTime=-1  MCHP_MASTERLINK=|  PinDigitalInput=[]  PinDigitalOutput=[]  PinAnalogInput=[]
      | AUAV_V3_TestSensors/Microchip Master
      | AUAV V3 Board
      | Busy Flag on D2 (RA6)
  Get WP from idx SIM : Subsystem
  WP Coord : Outport
  wires:
  Geod2LTP2/1 -> Environment Controller1/2
  Get WP Coord navsupport.c [updated 5.1.16]/1 -> Demux1/1
  Demux1/3 -> Geod2LTP2/5
  Demux1/2 -> Geod2LTP2/4
  Demux1/1 -> Geod2LTP2/3
  Get WP from idx SIM/1(Out1) -> Environment Controller1/1
  Environment Controller1/1 -> WP Coord/1
  GS R_in/1 -> Get WP from idx SIM/2(GS ECEF), Geod2LTP2/2
  GS LLA/1 -> Get WP from idx SIM/1(GS LLA), Geod2LTP2/1
  WP Idx/1 -> Get WP from idx SIM/3(idx), Get WP Coord navsupport.c [updated 5.1.16]/1

== system AUAV_V3_TestSensors/Inner Loop// Navigation/Navigation Encaps [updated 4.28.16]/Navigation/Normal WP Navigation/Get Frenet/get WP Coord from Index2 ==
  WP Idx : Inport
  GS LLA : Inport  Port=2
  GS R_in : Inport  Port=3
  Demux1 : Demux  Outputs=3
  Environment Controller1 : simulink/Signal Routing/Environment Controller
  Geod2LTP2 : SLUGS_Library/Navigation/Geod2LTP
  Get WP Coord navsupport.c [updated 5.1.16] : MCHP_Blockset/User Functions/C Function Call  ParseFilesChkbx=off  ListFunctions1=Custom Function  Function1=void getWP(unsigned char idx, float* WPpos)  AddHeaderDeclaration=on  Function1Type=when block is updated (default)  Fct1BlockIn=idx  FctReturnBlockOut=on  Fct1BlockOut=WPpos[3]  DataCollected=0  ORDERING=None  SampleTime=-1  MCHP_MASTERLINK=|  PinDigitalInput=[]  PinDigitalOutput=[]  PinAnalogInput=[]
      | AUAV_V3_TestSensors/Microchip Master
      | AUAV V3 Board
      | Busy Flag on D2 (RA6)
  Get WP from idx SIM : Subsystem
  WP Coord : Outport
  wires:
  Geod2LTP2/1 -> Environment Controller1/2
  Get WP Coord navsupport.c [updated 5.1.16]/1 -> Demux1/1
  Demux1/3 -> Geod2LTP2/5
  Demux1/2 -> Geod2LTP2/4
  Demux1/1 -> Geod2LTP2/3
  Get WP from idx SIM/1(Out1) -> Environment Controller1/1
  Environment Controller1/1 -> WP Coord/1
  GS R_in/1 -> Get WP from idx SIM/2(GS ECEF), Geod2LTP2/2
  GS LLA/1 -> Get WP from idx SIM/1(GS LLA), Geod2LTP2/1
  WP Idx/1 -> Get WP from idx SIM/3(idx), Get WP Coord navsupport.c [updated 5.1.16]/1

== system AUAV_V3_TestSensors/Inner Loop// Navigation/Navigation Encaps [updated 4.28.16]/Navigation/Normal WP Navigation/On WP Enable/Subsystem ==
  GS LLA : Inport
  GS R_in : Inport  Port=2
  Compute Frenet : Subsystem  AncestorBlock=SLUGS_Library/Navigation/Compute Frenet
  Constant : Constant  OutDataTypeStr=uint8  SampleTime=0.01
  Constant1 : Constant  Value=2  OutDataTypeStr=uint8  SampleTime=0.01
  GS LLA_1 : InportShadow
  GS R_in_1 : InportShadow  Port=2
  Terminator : Terminator
  get WP Coord from Index : Subsystem  AncestorBlock=SLUGS_Library/Navigation/get WP Coord from Index
  get WP Coord from Index1 : Subsystem  AncestorBlock=SLUGS_Library/Navigation/get WP Coord from Index
  WP0 : Outport
  T1 : Outport  Port=2
  wires:
  Constant/1 -> get WP Coord from Index/1(WP Idx)
  Compute Frenet/2(N) -> Terminator/1
  Compute Frenet/1(T) -> T1/1
  GS LLA/1 -> get WP Coord from Index/2(GS LLA)
  GS R_in/1 -> get WP Coord from Index/3(GS R_in)
  get WP Coord from Index/1(WP Coord) -> WP0/1, Compute Frenet/1(Pos 1)
  get WP Coord from Index1/1(WP Coord) -> Compute Frenet/2(Pos 2)
  Constant1/1 -> get WP Coord from Index1/1(WP Idx)
  GS LLA_1/1 -> get WP Coord from Index1/2(GS LLA)
  GS R_in_1/1 -> get WP Coord from Index1/3(GS R_in)

== system AUAV_V3_TestSensors/Inner Loop// Navigation/Navigation Encaps [updated 4.28.16]/Navigation/Normal WP Navigation/Vector Norm/dsPIC_SQRT ==
  x : Inport
  Environment Controller : simulink/Signal Routing/Environment Controller
  Math Function1 : Math  Operator=sqrt  SaturateOnIntegerOverflow=on
  mySqrt() apUtils.c [updated 5.1.16] : MCHP_Blockset/User Functions/C Function Call  ParseFilesChkbx=off  ListFunctions1=Custom Function  Function1=float mySqrt(float x)  AddHeaderDeclaration=on  Function1Type=when block is updated (default)  Fct1BlockIn=x  FctReturnBlockOut=on  DataCollected=0  ORDERING=None  SampleTime=-1  MCHP_MASTERLINK=|  PinDigitalInput=[]  PinDigitalOutput=[]  PinAnalogInput=[]
      | AUAV_V3_TestSensors/Microchip Master
      | AUAV V3 Board
      | Busy Flag on D2 (RA6)
  negprotect : MATLAB Function  TreatAsAtomicUnit=on
  sqrt(x) : Outport
  wires:
  x/1 -> negprotect/1(val)
  negprotect/1(zpVal) -> Math Function1/1, mySqrt() apUtils.c [updated 5.1.16]/1
  Environment Controller/1 -> sqrt(x)/1
  Math Function1/1 -> Environment Controller/1
  mySqrt() apUtils.c [updated 5.1.16]/1 -> Environment Controller/2

== system AUAV_V3_TestSensors/Inner Loop// Navigation/Navigation Encaps [updated 4.28.16]/Navigation/RTB//Follow Mobile Navigation/Vector Norm/dsPIC_SQRT ==
  x : Inport
  Environment Controller : simulink/Signal Routing/Environment Controller
  Math Function1 : Math  Operator=sqrt  SaturateOnIntegerOverflow=on
  mySqrt() apUtils.c [updated 5.1.16] : MCHP_Blockset/User Functions/C Function Call  ParseFilesChkbx=off  ListFunctions1=Custom Function  Function1=float mySqrt(float x)  AddHeaderDeclaration=on  Function1Type=when block is updated (default)  Fct1BlockIn=x  FctReturnBlockOut=on  DataCollected=0  ORDERING=None  SampleTime=-1  MCHP_MASTERLINK=|  PinDigitalInput=[]  PinDigitalOutput=[]  PinAnalogInput=[]
      | AUAV_V3_TestSensors/Microchip Master
      | AUAV V3 Board
      | Busy Flag on D2 (RA6)
  negprotect : MATLAB Function  TreatAsAtomicUnit=on
  sqrt(x) : Outport
  wires:
  x/1 -> negprotect/1(val)
  negprotect/1(zpVal) -> Math Function1/1, mySqrt() apUtils.c [updated 5.1.16]/1
  Environment Controller/1 -> sqrt(x)/1
  Math Function1/1 -> Environment Controller/1
  mySqrt() apUtils.c [updated 5.1.16]/1 -> Environment Controller/2

== system AUAV_V3_TestSensors/Inner Loop// Navigation/Navigation Encaps [updated 4.28.16]/Navigation/Recent Enable/Grab Upon Enable/Compute GS Location ==
  GS Location : Inport
  Demux : Demux  Outputs=3
  Geod2ECEF1 : Subsystem  mask{Re=6378137, Rp=6356752.3142}
      mask prompts: Re "Enter equatorial radius, m"; Rp "Enter polar radius,m"
  Mux1 : Mux  Inputs=2
  Mux2 : Mux  Inputs=3
  "Lon, Lat" : Outport
  R_in : Outport  Port=2
  wires:
  Mux2/1 -> R_in/1  "R_in"
  Mux1/1 -> "Lon, Lat"/1
  GS Location/1 -> Demux/1
  Demux/3 -> Mux1/1, Geod2ECEF1/3(lon,deg)
  Demux/2 -> Mux1/2, Geod2ECEF1/2("lat, deg")
  Demux/1 -> Geod2ECEF1/1("height, m")
  Geod2ECEF1/2("Ye, m ") -> Mux2/2
  Geod2ECEF1/1("Xe, m ") -> Mux2/1
  Geod2ECEF1/3("Ze, m ") -> Mux2/3

== system AUAV_V3_TestSensors/Inner Loop// Navigation/Navigation Encaps [updated 4.28.16]/Navigation/Recent Enable/Subsystem/Detect Rising Edge ==
  In1 : Inport
  Delay : Delay  DelayLength=1
  Logical Operator : Logic  AllPortsSameDT=off  OutDataTypeStr=boolean
  Relational Operator : RelationalOperator  Operator=~=  OutDataTypeStr=boolean
  Out1 : Outport
  wires:
  Delay/1 -> Relational Operator/1
  Relational Operator/1 -> Logical Operator/1
  In1/1 -> Delay/1, Relational Operator/2, Logical Operator/2
  Logical Operator/1 -> Out1/1

== system AUAV_V3_TestSensors/Position_and_Attitude_Filter/Position Filter/BlendPosVel/CompFiltRate/1D Filter1/Filter2 ==
  In1 : Inport
  Discrete Zero-Pole : DiscreteZeroPole  Zeros=zerosd  Poles=polesd  Gain=gaind  SampleTime=SampleTime
  Out1 : Outport
  wires:
  Discrete Zero-Pole/1 -> Out1/1
  In1/1 -> Discrete Zero-Pole/1

== system AUAV_V3_TestSensors/Position_and_Attitude_Filter/Position Filter/BlendPosVel/CompFiltRate1/1D Filter1/Filter2 ==
  In1 : Inport
  Discrete Zero-Pole : DiscreteZeroPole  Zeros=zerosd  Poles=polesd  Gain=gaind  SampleTime=SampleTime
  Out1 : Outport
  wires:
  Discrete Zero-Pole/1 -> Out1/1
  In1/1 -> Discrete Zero-Pole/1

== system AUAV_V3_TestSensors/Position_and_Attitude_Filter/Position Filter/BlendPosVel/CompRateOnly/1D Filter1/Filter2 ==
  In1 : Inport
  Discrete Zero-Pole : DiscreteZeroPole  Zeros=zerosd  Poles=polesd  Gain=gaind  SampleTime=SampleTime
  Out1 : Outport
  wires:
  Discrete Zero-Pole/1 -> Out1/1
  In1/1 -> Discrete Zero-Pole/1

== system AUAV_V3_TestSensors/Sensor_Data_Adapter/Sensor Suite/Low Pass Filtering,Temperature Compensation and Calibration/Baro Altimeter/Initial Baro Bias/Low Pass8 ==
  In1 : Inport
  Discrete Zero-Pole : DiscreteZeroPole  Zeros=zerosd  Poles=polesd  Gain=gaind  SampleTime=SampleTime
  Out1 : Outport
  wires:
  In1/1 -> Discrete Zero-Pole/1
  Discrete Zero-Pole/1 -> Out1/1

== system AUAV_V3_TestSensors/Inner Loop// Navigation/Navigation Encaps [updated 4.28.16]/Navigation/Circle Navigation/Intersection. Circular Navigation/Compute Angle Between Vectors1/Vector Norm ==
  Vector : Inport
  dsPIC Dot Product : SLUGS_Library/dsPIC Dot Product
  dsPIC_SQRT : Subsystem  AncestorBlock=SLUGS_Library/dsPIC_SQRT
  Norm : Outport
  wires:
  dsPIC_SQRT/1(sqrt(x)) -> Norm/1
  Vector/1 -> dsPIC Dot Product/2, dsPIC Dot Product/1
  dsPIC Dot Product/1 -> dsPIC_SQRT/1(x)

== system AUAV_V3_TestSensors/Inner Loop// Navigation/Navigation Encaps [updated 4.28.16]/Navigation/Circle Navigation/Intersection. Circular Navigation/Compute Angle Between Vectors1/dsPIC_acos ==
  x : Inport
  Environment Controller : simulink/Signal Routing/Environment Controller
  Trigonometric Function : Trigonometry  Operator=acos
  myAcos() apUtils.c [updated 5.1.16] : MCHP_Blockset/User Functions/C Function Call  ParseFilesChkbx=off  ListFunctions1=Custom Function  Function1=float myAcos(float x)  AddHeaderDeclaration=on  Function1Type=when block is updated (default)  Fct1BlockIn=x  FctReturnBlockOut=on  ORDERING=None  SampleTime=-1  MCHP_MASTERLINK=|  PinDigitalInput=[]  PinDigitalOutput=[]  PinAnalogInput=[]
      | AUAV_V3_TestSensors/Microchip Master
      | AUAV V3 Board
      | Busy Flag on D2 (RA6)
  acos(x) : Outport
  wires:
  Environment Controller/1 -> acos(x)/1
  myAcos() apUtils.c [updated 5.1.16]/1 -> Environment Controller/2
  Trigonometric Function/1 -> Environment Controller/1
  x/1 -> Trigonometric Function/1, myAcos() apUtils.c [updated 5.1.16]/1

== system AUAV_V3_TestSensors/Inner Loop// Navigation/Navigation Encaps [updated 4.28.16]/Navigation/Circle Navigation/Intersection. Circular Navigation/Compute Angle Between Vectors2/Vector Norm ==
  Vector : Inport
  dsPIC Dot Product : SLUGS_Library/dsPIC Dot Product
  dsPIC_SQRT : Subsystem  AncestorBlock=SLUGS_Library/dsPIC_SQRT
  Norm : Outport
  wires:
  dsPIC_SQRT/1(sqrt(x)) -> Norm/1
  Vector/1 -> dsPIC Dot Product/2, dsPIC Dot Product/1
  dsPIC Dot Product/1 -> dsPIC_SQRT/1(x)

== system AUAV_V3_TestSensors/Inner Loop// Navigation/Navigation Encaps [updated 4.28.16]/Navigation/Circle Navigation/Intersection. Circular Navigation/Compute Angle Between Vectors2/dsPIC_acos ==
  x : Inport
  Environment Controller : simulink/Signal Routing/Environment Controller
  Trigonometric Function : Trigonometry  Operator=acos
  myACos() apUtils.c [updated 5.1.16] : MCHP_Blockset/User Functions/C Function Call  ParseFilesChkbx=off  ListFunctions1=Custom Function  Function1=float myAcos(float x)  AddHeaderDeclaration=on  Function1Type=when block is updated (default)  Fct1BlockIn=x  FctReturnBlockOut=on  ORDERING=None  SampleTime=-1  MCHP_MASTERLINK=|  PinDigitalInput=[]  PinDigitalOutput=[]  PinAnalogInput=[]
      | AUAV_V3_TestSensors/Microchip Master
      | AUAV V3 Board
      | Busy Flag on D2 (RA6)
  acos(x) : Outport
  wires:
  Environment Controller/1 -> acos(x)/1
  myACos() apUtils.c [updated 5.1.16]/1 -> Environment Controller/2
  Trigonometric Function/1 -> Environment Controller/1
  x/1 -> Trigonometric Function/1, myACos() apUtils.c [updated 5.1.16]/1

== system AUAV_V3_TestSensors/Inner Loop// Navigation/Navigation Encaps [updated 4.28.16]/Navigation/L2+/Get Sin, Cos eta/Get Groundspeed/Vector Norm ==
  Vector : Inport
  dsPIC Dot Product : SLUGS_Library/dsPIC Dot Product
  dsPIC_SQRT : Subsystem  AncestorBlock=SLUGS_Library/dsPIC_SQRT
  Norm : Outport
  wires:
  dsPIC_SQRT/1(sqrt(x)) -> Norm/1
  Vector/1 -> dsPIC Dot Product/2, dsPIC Dot Product/1
  dsPIC Dot Product/1 -> dsPIC_SQRT/1(x)

== system AUAV_V3_TestSensors/Inner Loop// Navigation/Navigation Encaps [updated 4.28.16]/Navigation/Normal WP Navigation/Compute WP Switching Trigger/Compute Projection/Protect NaNs ==
  In1 : Inport
  Integer Delay3 : Delay  DelayLength=1  InputProcessing=Inherited  SampleTime=T
  Relational Operator2 : RelationalOperator  Operator===  OutDataTypeStr=uint(8)
  Switch3 : Switch  Criteria=u2 > Threshold  Threshold=0.3  SampleTime=.01
  Out1 : Outport
  wires:
  Relational Operator2/1 -> Switch3/2
  In1/1 -> Switch3/1, Relational Operator2/1, Relational Operator2/2
  Switch3/1 -> Integer Delay3/1, Out1/1
  Integer Delay3/1 -> Switch3/3

== system AUAV_V3_TestSensors/Inner Loop// Navigation/Navigation Encaps [updated 4.28.16]/Navigation/Normal WP Navigation/Get Frenet/Compute Frenet/Normalize Vector ==
  Vector : Inport
  Divide : Product  Inputs=*/
  Vector Norm : Subsystem  AncestorBlock=SLUGS_Library/Vector Norm
  Zero Bound : Saturate  UpperLimit=inf  LowerLimit=0.001
  Normalized : Outport
  wires:
  Vector/1 -> Vector Norm/1(Vector), Divide/1
  Vector Norm/1(Norm) -> Zero Bound/1
  Zero Bound/1 -> Divide/2
  Divide/1 -> Normalized/1

== system AUAV_V3_TestSensors/Inner Loop// Navigation/Navigation Encaps [updated 4.28.16]/Navigation/Normal WP Navigation/Get Frenet/Compute Frenet/Normalize Vector  ==
  Vector : Inport
  Divide : Product  Inputs=*/
  Vector Norm : Subsystem  AncestorBlock=SLUGS_Library/Vector Norm
  Zero Bound : Saturate  UpperLimit=inf  LowerLimit=0.001
  Normalized : Outport
  wires:
  Vector/1 -> Vector Norm/1(Vector), Divide/1
  Vector Norm/1(Norm) -> Zero Bound/1
  Zero Bound/1 -> Divide/2
  Divide/1 -> Normalized/1

== system AUAV_V3_TestSensors/Inner Loop// Navigation/Navigation Encaps [updated 4.28.16]/Navigation/Normal WP Navigation/Get Frenet/get WP Coord from Index1/Get WP from idx SIM ==
  GS LLA : Inport
  GS ECEF : Inport  Port=2
  idx : Inport  Port=3
  Constant : Constant  Value=latlong_WP  OutDataTypeStr=uint8  SampleTime=0.01
  Constant1 : Constant  Value=Ypoints  OutDataTypeStr=double  SampleTime=0.01
  Constant2 : Constant  Value=Xpoints  OutDataTypeStr=double  SampleTime=0.01
  Constant3 : Constant  Value=Zpoints  OutDataTypeStr=double  SampleTime=0.01
  Data Type Conversion : DataTypeConversion  OutDataTypeStr=double
  Data Type Conversion1 : DataTypeConversion  OutDataTypeStr=single
  Demux : Demux  Outputs=3
  Geod2LTP1 : SLUGS_Library/Navigation/Geod2LTP
  Mux : Mux  Inputs=3
  Switch : Switch  Criteria=u2 > Threshold  Threshold=0.3  ZeroCross=off
  Zero out Z1 : MATLAB Function  TreatAsAtomicUnit=on
  Zero out Z2 : MATLAB Function  TreatAsAtomicUnit=on
  Zero out Z3 : MATLAB Function  TreatAsAtomicUnit=on
  Out1 : Outport
  wires:
  Constant2/1 -> Zero out Z2/2(vect)
  Constant3/1 -> Zero out Z3/2(vect)
  Constant1/1 -> Zero out Z1/2(vect)
  Switch/1 -> Out1/1
  idx/1 -> Data Type Conversion/1
  GS ECEF/1 -> Geod2LTP1/2
  GS LLA/1 -> Geod2LTP1/1
  Data Type Conversion1/1 -> Demux/1, Switch/3
  Geod2LTP1/1 -> Switch/1
  Demux/3 -> Geod2LTP1/5
  Demux/2 -> Geod2LTP1/4
  Demux/1 -> Geod2LTP1/3
  Constant/1 -> Switch/2
  Mux/1 -> Data Type Conversion1/1
  Zero out Z3/1(y) -> Mux/3
  Zero out Z1/1(y) -> Mux/2
  Zero out Z2/1(y) -> Mux/1
  Data Type Conversion/1 -> Zero out Z3/1(idx), Zero out Z1/1(idx), Zero out Z2/1(idx)

== system AUAV_V3_TestSensors/Inner Loop// Navigation/Navigation Encaps [updated 4.28.16]/Navigation/Normal WP Navigation/Get Frenet/get WP Coord from Index2/Get WP from idx SIM ==
  GS LLA : Inport
  GS ECEF : Inport  Port=2
  idx : Inport  Port=3
  Constant : Constant  Value=latlong_WP  OutDataTypeStr=uint8  SampleTime=0.01
  Constant1 : Constant  Value=Ypoints  OutDataTypeStr=double  SampleTime=0.01
  Constant2 : Constant  Value=Xpoints  OutDataTypeStr=double  SampleTime=0.01
  Constant3 : Constant  Value=Zpoints  OutDataTypeStr=double  SampleTime=0.01
  Data Type Conversion : DataTypeConversion  OutDataTypeStr=double
  Data Type Conversion1 : DataTypeConversion  OutDataTypeStr=single
  Demux : Demux  Outputs=3
  Geod2LTP1 : SLUGS_Library/Navigation/Geod2LTP
  Mux : Mux  Inputs=3
  Switch : Switch  Criteria=u2 > Threshold  Threshold=0.3  ZeroCross=off
  Zero out Z1 : MATLAB Function  TreatAsAtomicUnit=on
  Zero out Z2 : MATLAB Function  TreatAsAtomicUnit=on
  Zero out Z3 : MATLAB Function  TreatAsAtomicUnit=on
  Out1 : Outport
  wires:
  Constant2/1 -> Zero out Z2/2(vect)
  Constant3/1 -> Zero out Z3/2(vect)
  Constant1/1 -> Zero out Z1/2(vect)
  Switch/1 -> Out1/1
  idx/1 -> Data Type Conversion/1
  GS ECEF/1 -> Geod2LTP1/2
  GS LLA/1 -> Geod2LTP1/1
  Data Type Conversion1/1 -> Demux/1, Switch/3
  Geod2LTP1/1 -> Switch/1
  Demux/3 -> Geod2LTP1/5
  Demux/2 -> Geod2LTP1/4
  Demux/1 -> Geod2LTP1/3
  Constant/1 -> Switch/2
  Mux/1 -> Data Type Conversion1/1
  Zero out Z3/1(y) -> Mux/3
  Zero out Z1/1(y) -> Mux/2
  Zero out Z2/1(y) -> Mux/1
  Data Type Conversion/1 -> Zero out Z3/1(idx), Zero out Z1/1(idx), Zero out Z2/1(idx)

== system AUAV_V3_TestSensors/Inner Loop// Navigation/Navigation Encaps [updated 4.28.16]/Navigation/Normal WP Navigation/On WP Enable/Subsystem/Compute Frenet ==
  Pos 1 : Inport
  Pos 2 : Inport  Port=2
  Add : Sum  Inputs=-+
  Normalize Vector : Subsystem  AncestorBlock=SLUGS_Library/Navigation/Normalize Vector
  "Normalize Vector " : Subsystem  AncestorBlock=SLUGS_Library/Navigation/Normalize Vector
  Select N Terms : MATLAB Function  TreatAsAtomicUnit=on
  T : Outport
  N : Outport  Port=2
  wires:
  "Normalize Vector "/1(Normalized) -> N/1
  Select N Terms/1(N) -> "Normalize Vector "/1(Vector)
  Normalize Vector/1(Normalized) -> Select N Terms/1(T), T/1
  Add/1 -> Normalize Vector/1(Vector)
  Pos 2/1 -> Add/2
  Pos 1/1 -> Add/1

== system AUAV_V3_TestSensors/Inner Loop// Navigation/Navigation Encaps [updated 4.28.16]/Navigation/Normal WP Navigation/On WP Enable/Subsystem/get WP Coord from Index ==
  WP Idx : Inport
  GS LLA : Inport  Port=2
  GS R_in : Inport  Port=3
  Demux1 : Demux  Outputs=3
  Environment Controller1 : simulink/Signal Routing/Environment Controller
  Geod2LTP2 : SLUGS_Library/Navigation/Geod2LTP
  Get WP Coord navsupport.c [updated 5.1.16] : MCHP_Blockset/User Functions/C Function Call  ParseFilesChkbx=off  ListFunctions1=Custom Function  Function1=void getWP(unsigned char idx, float* WPpos)  AddHeaderDeclaration=on  Function1Type=when block is updated (default)  Fct1BlockIn=idx  FctReturnBlockOut=on  Fct1BlockOut=WPpos[3]  DataCollected=0  ORDERING=None  SampleTime=-1  MCHP_MASTERLINK=|  PinDigitalInput=[]  PinDigitalOutput=[]  PinAnalogInput=[]
      | AUAV_V3_TestSensors/Microchip Master
      | AUAV V3 Board
      | Busy Flag on D2 (RA6)
  Get WP from idx SIM : Subsystem
  WP Coord : Outport
  wires:
  Geod2LTP2/1 -> Environment Controller1/2
  Get WP Coord navsupport.c [updated 5.1.16]/1 -> Demux1/1
  Demux1/3 -> Geod2LTP2/5
  Demux1/2 -> Geod2LTP2/4
  Demux1/1 -> Geod2LTP2/3
  Get WP from idx SIM/1(Out1) -> Environment Controller1/1
  Environment Controller1/1 -> WP Coord/1
  GS R_in/1 -> Get WP from idx SIM/2(GS ECEF), Geod2LTP2/2
  GS LLA/1 -> Get WP from idx SIM/1(GS LLA), Geod2LTP2/1
  WP Idx/1 -> Get WP from idx SIM/3(idx), Get WP Coord navsupport.c [updated 5.1.16]/1
